simulink model "Planta"  (R2026a)
settings: Solver=VariableStepAuto
settings Model: Creator=Yahoff  LastModifiedBy=Yahoff

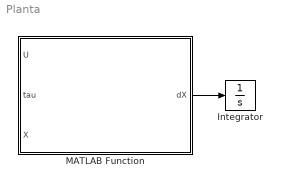
== system Planta ==
  Integrator : Integrator  InitialCondition=[0;0;0;0;0;0]
  MATLAB Function : MATLAB Function  TreatAsAtomicUnit=on
  wires:
  MATLAB Function/1(dX) -> Integrator/1

== matlab function Planta/MATLAB Function ==
  data: U input; dX output; tau input; X input
function dX = planta(U, tau, X)

    m = 1; J = 1; g = 9.81;

    x     = X(1);
    xdot  = X(2);
    z     = X(3);
    zdot  = X(4);
    th    = X(5);
    thdot = X(6);

    xdd  = -(U/m)*sin(th);
    zdd  =  (U/m)*cos(th) - g;
    thdd =  tau/J;

    dX = [xdot; xdd; zdot; zdd; thdot; thdd];
